simulink model "model"  (R2020b)
settings: Solver=ode113  StartTime=0.0  StopTime=200  MaxStep=0.2  RelTol=1e-8  AbsTol=1e-8
values from neighbouring files (symbols this model uses):
  data = struct()    [config.m]
libraries: libraryMatlab x7
settings Model: Creator=pacif  LastModifiedBy=pacif

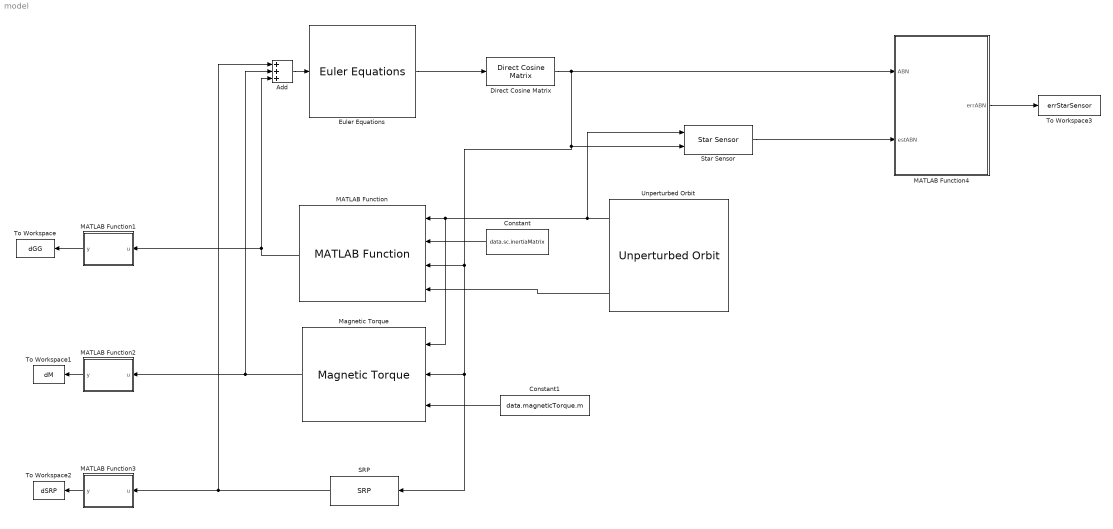
== system model ==
  Add : Sum  Inputs=+++
  Constant : Constant  Value=data.sc.inertiaMatrix
  Constant1 : Constant  Value=data.magneticTorque.m
  Direct Cosine Matrix : libraryMatlab/Direct Cosine Matrix  SystemSampleTime=-1  VariantActivationTime=update diagram  Latency=0  AutoFrameSizeCalculation=off
  Euler Equations : libraryMatlab/Euler Equations  SystemSampleTime=-1  VariantActivationTime=update diagram  Latency=0  AutoFrameSizeCalculation=off
  MATLAB Function : libraryMatlab/MATLAB Function  SystemSampleTime=-1  VariantActivationTime=update diagram  Latency=0  AutoFrameSizeCalculation=off
  MATLAB Function1 : MATLAB Function  TreatAsAtomicUnit=on
  MATLAB Function2 : MATLAB Function  TreatAsAtomicUnit=on
  MATLAB Function3 : MATLAB Function  TreatAsAtomicUnit=on
  MATLAB Function4 : MATLAB Function  TreatAsAtomicUnit=on
  Magnetic Torque : libraryMatlab/Magnetic Torque  SystemSampleTime=-1  VariantActivationTime=update diagram  Latency=0  AutoFrameSizeCalculation=off
  SRP : libraryMatlab/SRP  SystemSampleTime=-1  VariantActivationTime=update diagram  Latency=0  AutoFrameSizeCalculation=off
  Star Sensor : libraryMatlab/Star Sensor  SystemSampleTime=-1  VariantActivationTime=update diagram  Latency=0  AutoFrameSizeCalculation=off
  To Workspace : ToWorkspace  VariableName=dGG  SaveFormat=Timeseries  SampleTime=-1
  To Workspace1 : ToWorkspace  VariableName=dM  SaveFormat=Timeseries  SampleTime=-1
  To Workspace2 : ToWorkspace  VariableName=dSRP  SaveFormat=Timeseries  SampleTime=-1
  To Workspace3 : ToWorkspace  VariableName=errStarSensor  SaveFormat=Timeseries  SampleTime=-1
  Unperturbed Orbit : libraryMatlab/Unperturbed Orbit  SystemSampleTime=-1  VariantActivationTime=update diagram  Latency=0  AutoFrameSizeCalculation=off
  wires:
  Euler Equations/1 -> Direct Cosine Matrix/1
  Direct Cosine Matrix/1 -> MATLAB Function4/1(ABN), Star Sensor/2, SRP/1, Magnetic Torque/2, MATLAB Function/3
  Unperturbed Orbit/3 -> MATLAB Function/4
  Unperturbed Orbit/1 -> Star Sensor/1, Magnetic Torque/1, MATLAB Function/1
  Constant/1 -> MATLAB Function/2
  Add/1 -> Euler Equations/1
  MATLAB Function/1 -> MATLAB Function1/1(u), Add/3
  Constant1/1 -> Magnetic Torque/3
  Magnetic Torque/1 -> MATLAB Function2/1(u), Add/2
  SRP/1 -> MATLAB Function3/1(u), Add/1
  MATLAB Function3/1(y) -> To Workspace2/1
  MATLAB Function2/1(y) -> To Workspace1/1
  MATLAB Function1/1(y) -> To Workspace/1
  Star Sensor/1 -> MATLAB Function4/2(estABN)
  MATLAB Function4/1(errABN) -> To Workspace3/1

== matlab function model/MATLAB Function1 ==
  data: u input; y output
function y = normFun(u)

y = norm(u);

== matlab function model/MATLAB Function3 ==
  data: u input; y output
function y = normFun(u)

y = norm(u);

== matlab function model/MATLAB Function4 ==
  data: ABN input; errABN output; estABN input
function errABN = errorABN(ABN,estABN)

errMAT = abs(ABN - estABN);

errABN = max(errMAT(:));

== matlab function model/MATLAB Function2 ==
  data: u input; y output
function y = normFun(u)

y = norm(u);
